simulink model "part_c"  (R2017b)
settings: Solver=VariableStepAuto  StartTime=0.0  StopTime=10.0  RelTol=1e-3
values from neighbouring files (symbols this model uses):
  a = [0 1;-1 -0.7]    [P2a.m]    (also in P2b.m; P2c.m)
  b = [0;1]    [P2a.m]    (also in P2b.m; P2c.m)
  c = [1 0;0 0]    [P2a.m]    (also in P2b.m; P2c.m = [1 0)
  P0 = 100*eye(2)    [P2c.m]
undefined symbols (not defined in the file or in its folder): K, l
settings Model: Creator=Soutrik  LastModifiedBy=Soutrik

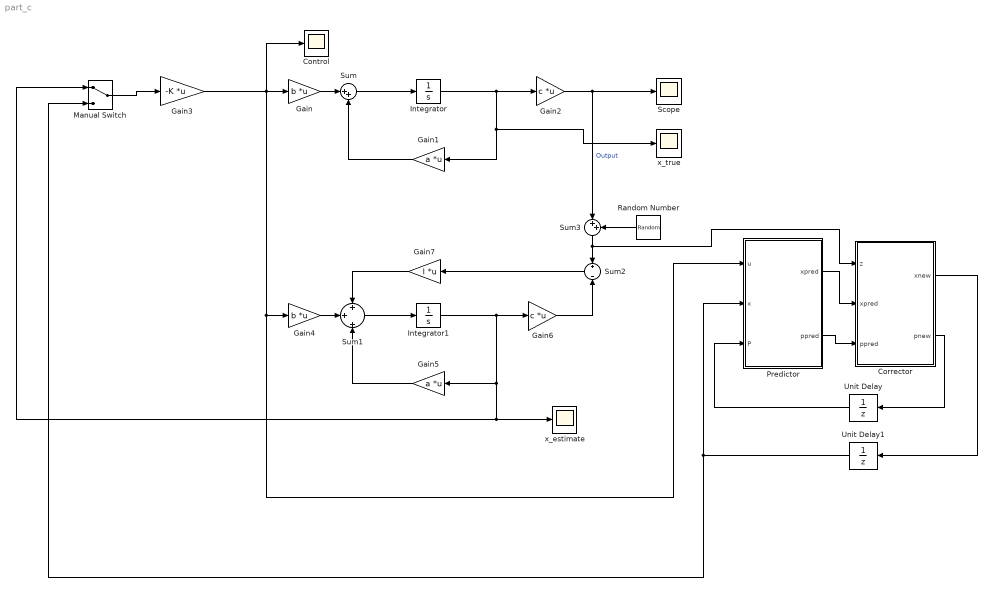
== system part_c ==
  Control : Scope
  Corrector : MATLAB Function  TreatAsAtomicUnit=on
  Gain : Gain  Gain=b  Multiplication=Matrix(K*u)
  Gain1 : Gain  Gain=a  Multiplication=Matrix(K*u)
  Gain2 : Gain  Gain=c  Multiplication=Matrix(K*u)
  Gain3 : Gain  Gain=-K  Multiplication=Matrix(K*u)
  Gain4 : Gain  Gain=b  Multiplication=Matrix(K*u)
  Gain5 : Gain  Gain=a  Multiplication=Matrix(K*u)
  Gain6 : Gain  Gain=c  Multiplication=Matrix(K*u)
  Gain7 : Gain  Gain=l  Multiplication=Matrix(K*u)
  Integrator : Integrator  InitialCondition=[1 0]
  Integrator1 : Integrator  InitialCondition=[1 0]
  Manual Switch : ManualSwitch
  Predictor : MATLAB Function  TreatAsAtomicUnit=on
  Random Number : RandomNumber  Variance=0.1  Seed=5  SampleTime=0.01
  Scope : Scope
  Sum : Sum  Inputs=|++
  Sum1 : Sum  Inputs=+|+|+
  Sum2 : Sum  Inputs=+||-
  Sum3 : Sum  Inputs=|++
  Unit Delay : UnitDelay  InitialCondition=P0  SampleTime=-1
  Unit Delay1 : UnitDelay  InitialCondition=[1 0]  SampleTime=-1
  x_estimate : Scope
  x_true : Scope
  wires:
  Integrator/1 -> x_true/1, Gain1/1, Gain2/1
  Gain4/1 -> Sum1/2
  Integrator1/1 -> Gain5/1, x_estimate/1, Manual Switch/1, Gain6/1
  Random Number/1 -> Sum3/2
  Sum3/1 -> Corrector/1(z), Sum2/1
  Gain7/1 -> Sum1/1
  Sum2/1 -> Gain7/1
  Gain5/1 -> Sum1/3
  Sum1/1 -> Integrator1/1
  Sum/1 -> Integrator/1
  Gain6/1 -> Sum2/2
  Gain3/1 -> Predictor/1(u), Gain4/1, Gain/1, Control/1
  Gain1/1 -> Sum/2
  Gain2/1 -> Scope/1, Sum3/1  "Output"
  Gain/1 -> Sum/1
  Manual Switch/1 -> Gain3/1
  Predictor/2(ppred) -> Corrector/3(ppred)
  Predictor/1(xpred) -> Corrector/2(xpred)
  Corrector/2(pnew) -> Unit Delay/1
  Unit Delay/1 -> Predictor/3(P)
  Unit Delay1/1 -> Manual Switch/2, Predictor/2(x)
  Corrector/1(xnew) -> Unit Delay1/1

== matlab function part_c/Corrector ==
  data: z input size=4; xpred input size=[4 1]; xnew output size=4; ppred input size=[4 4]; pnew output size=[4 4]
%% Corrector algorithm
function [xnew,pnew]= corrector(z, xpred, ppred)
R=0.0001*eye(4);
%R = eye(4);
C = [ 1.0000 -0.0050 0.0000 0.0000;
    0.0000 1.0025 0.0000 -0.0000;
    0.1604 0.0084 0.9612 0.2769;
    0.0000 -0.0049 -0.0011 0.0040 ];
H=C;
k=ppred*H'*inv((H*ppred*H')+R);
pnew=((eye(4)-k*H)*ppred*transpose(eye(4)-k*H))+k*R*k';
xnew=xpred+k*(z-H*xpred);
end

== matlab function part_c/Predictor ==
  data: u input size=2; xpred output size=4; x input size=4; ppred output size=[4 4]; P input size=[4 4]
%% Predictor algorithm
function [xpred, ppred]= predictor(u,x,P)
a = [ -0.0000 1.0000 -0.0000 -0.0000;
    -0.0000 -0.5004 -0.0022 0.0064;
    -30.8405 -66.2409 0.0089 0.0199;
    -8.8533 224.6563 -0.0360 -0.8097 ];

b = [ -0.0000 0.0000;
    -0.0226 0.0212;
    0.0010 0.0035;
    -0.1601 0.2148 ];
Q=10*eye(4);
R=eye(2);

ad=expm(a*0.01);
bd=inv(a)*(ad-eye(4))*b;

F=[-a Q;zeros(4,4) a'];
G=expm(F*0.01);
Glr=G(5:8,5:8);
Gur=G(1:4,5:8);
Qd=Glr'*Gur;

xpred=ad*x+bd*u;
ppred=ad*P+ad'*Qd;
end
